simulink model "FuzzyPD_Ship"  (Simulink 8.8)
settings: Solver=ode5  StartTime=0.0  StopTime=4000  FixedStep=0.1  MaxStep=0.1  RelTol=1e-3
PreLoadFcn:
  | FuzzyPD=readfis('FuzzyPD_Ship.fis');
StartFcn:
  | FuzzyPD=readfis('FuzzyPD_Ship.fis');
undefined symbols (not defined in the file or in its folder): sigbuilder_block
libraries: fuzblock x1
settings Model: Creator=Huynh Thai Hoang  LastModifiedBy=HTH  ExtModeTrigMode=oneshot  ExtModeArmWhenConnect=off
settings SolverCC: InitialStep=0.1
settings DataIOCC: LimitDataPoints=off  SaveOutput=off  SaveTime=off  SignalLoggingName=sigsOut
settings OptimizationCC: BooleanDataType=off  ExpressionDepthLimit=2147483647
settings DebuggingCC: SaveWithParameterizedLinksMsg=none  SignalResolutionControl=TryResolveAllWithWarning  MultiTaskDSMMsg=warning  MultiTaskCondExecSysMsg=none
settings HardwareCC: TargetUnknown=on

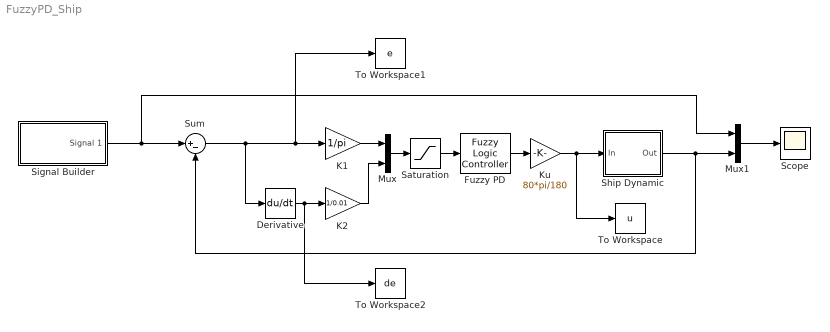
== system FuzzyPD_Ship ==
  Derivative : Derivative
  Fuzzy PD : fuzblock/Fuzzy Logic  Controller  fis=FuzzyPD
  K1 : Gain  Gain=1/pi  SaturateOnIntegerOverflow=on  OutDataTypeStr=Inherit: Same as input  ParamDataTypeStr=Inherit: Same as input
  K2 : Gain  Gain=1/0.01  SaturateOnIntegerOverflow=on  OutDataTypeStr=Inherit: Same as input  ParamDataTypeStr=Inherit: Same as input
  Ku : Gain  Gain=80*pi/180  SaturateOnIntegerOverflow=on  OutDataTypeStr=Inherit: Same as input  ParamDataTypeStr=Inherit: Same as input
  Mux : Mux  Inputs=2
  Mux1 : Mux  Inputs=2
  Saturation : Saturate  UpperLimit=1  LowerLimit=-1
  Scope : Scope
  Ship Dynamic : Subsystem
      mask init:
      | L=161;V=5;
      | k0=-3.86;T10=5.66; T20=0.38;T30=0.89;
      | k=k0*V/L;
      | T1=T10*L/V;
      | T2=T20*L/V;
      | T3=T30*L/V;
      mask Display:
      | plot([0.1 0.3 0.7 0.9 0.1],[0.3 0.1 0.1 0.3 0.3]);
      | plot([0.3 0.3 0.7 0.7],[0.3 0.5 0.5 0.3]);
      | plot([0.5 0.5 0.3 0.5],[0.5 0.9 0.7 0.7])
  Signal Builder : Subsystem  Tag=STV Subsys  LoadFcn=sigbuilder_block('load',[437.25 153 550.5 359.25 ]);  StartFcn=sigbuilder_block('start');  StopFcn=sigbuilder_block('stop');  ClipboardFcn=sigbuilder_block('clipboard');  mask(Sigbuilder block){tuvar=[0:10]}
      mask help: Simulink:masks:SigbuilderBlock_MD
      mask init:
      | if ~strcmp(get_param(bdroot(gcbh),'SimulationStatus'),'stopped') tuvar = sigbuilder_block('maskInit'); end
      settings: CopyFcn=sigbuilder_block('copy');  DeleteFcn=sigbuilder_block('delete');  ModelCloseFcn=sigbuilder_block('modelClose');  PreSaveFcn=sigbuilder_block('preSave');  PauseFcn=sigbuilder_block('pause');  ContinueFcn=sigbuilder_block('continue');  NameChangeFcn=sigbuilder_block('namechange');  OpenFcn=sigbuilder_block('open',[437.6 199.2 550.4 400 ]);  CloseFcn=sigbuilder_block('close');
      mask Display: plot(0, 0, 100, 100,[2, 2, 32, 32, 2], [68, 8, 8, 68, 68],[32, 2], [38, 38], [32, 19, 2],[53, 60, 44], [32, 17, 17, 2],[16, 16, 31, 31]);txt = getActiveGroup(gcbh);text(2, 100, txt,'verticalAlignment', 'top');
  Sum : Sum  Inputs=|+-  SaturateOnIntegerOverflow=on
  To Workspace : ToWorkspace  VariableName=u  SampleTime=-1
  To Workspace1 : ToWorkspace  VariableName=e  SampleTime=-1
  To Workspace2 : ToWorkspace  VariableName=de  SampleTime=-1
  wires:
  Ship Dynamic/1(Out) -> Sum/2, Mux1/2
  Sum/1 -> To Workspace1/1, K1/1, Derivative/1
  Derivative/1 -> To Workspace2/1, K2/1
  K1/1 -> Mux/1
  K2/1 -> Mux/2
  Mux/1 -> Saturation/1
  Fuzzy PD/1 -> Ku/1
  Ku/1 -> To Workspace/1, Ship Dynamic/1(In)
  Saturation/1 -> Fuzzy PD/1
  Mux1/1 -> Scope/1
  Signal Builder/1(Signal 1) -> Sum/1, Mux1/1

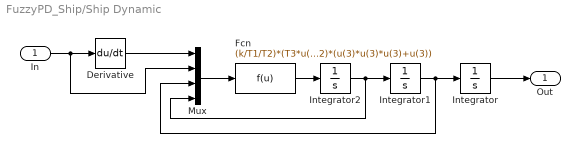
== system FuzzyPD_Ship/Ship Dynamic ==
  In : Inport
  Derivative : Derivative
  Fcn : Fcn  Expr=(k/T1/T2)*(T3*u(1)+u(2))-(1/T1+1/T2)*u(4)-(1/T1/T2)*(u(3)*u(3)*u(3)+u(3))
  Integrator : Integrator
  Integrator1 : Integrator
  Integrator2 : Integrator
  Mux : Mux
  Out : Outport
  wires:
  Mux/1 -> Fcn/1
  Derivative/1 -> Mux/1
  Fcn/1 -> Integrator2/1
  In/1 -> Mux/2, Derivative/1
  Integrator2/1 -> Mux/4, Integrator1/1
  Integrator1/1 -> Mux/3, Integrator/1
  Integrator/1 -> Out/1

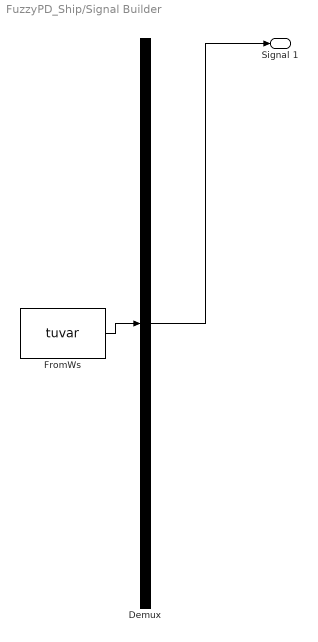
== system FuzzyPD_Ship/Signal Builder ==
  Demux : Demux  Tag=STV Demux  Outputs=1
  FromWs : FromWorkspace  Tag=STV FromWs  VariableName=tuvar  SampleTime=0  SigBuilderData=DataTag0  VnvData=DataTag1
      SigBuilderData=|
      | common.afterFinalStr = 'Extrapolate'
      | common.sampleTime = 0
      | dataSet.timeRange = [0 4000]
      | dataSet.name = 'Group 1'
      | sbobj.Groups.Name = 'Group 1'
      | sbobj.Groups.Signals.Name = 'Signal 1'
      | sbobj.Groups.Signals.XData = [0 1000 1000 2010 2010 3000 3000 4000]
      | sbobj.Groups.Signals.YData = [0.595 0.595 -0.48 -0.48 0.48 0.48 0 0]
      | sbobj.Groups.TimeRange = [0 4000]
  Signal 1 : Outport  Tag=STV Outport
  wires:
  Demux/1 -> Signal 1/1
  FromWs/1 -> Demux/1
